simulink model "ExtensionSimulation2CONT"  (R2015b)
settings: Solver=VariableStepAuto  StartTime=0.0  StopTime=60  RelTol=1e-3
values from neighbouring files (symbols this model uses):
  beta_str = 0.5*ones(1,10)    [PlotChannelCont.m]
undefined symbols (not defined in the file or in its folder): alpha_str, MemoryGain, nu_pc, sigbuilder_block, teta, w_e, w_g, w_minus, w_pc, w_plus, w_s, w_t
libraries: fuzblock x35, simulink x1
settings Model: Creator=acaso  LastModifiedBy=acaso

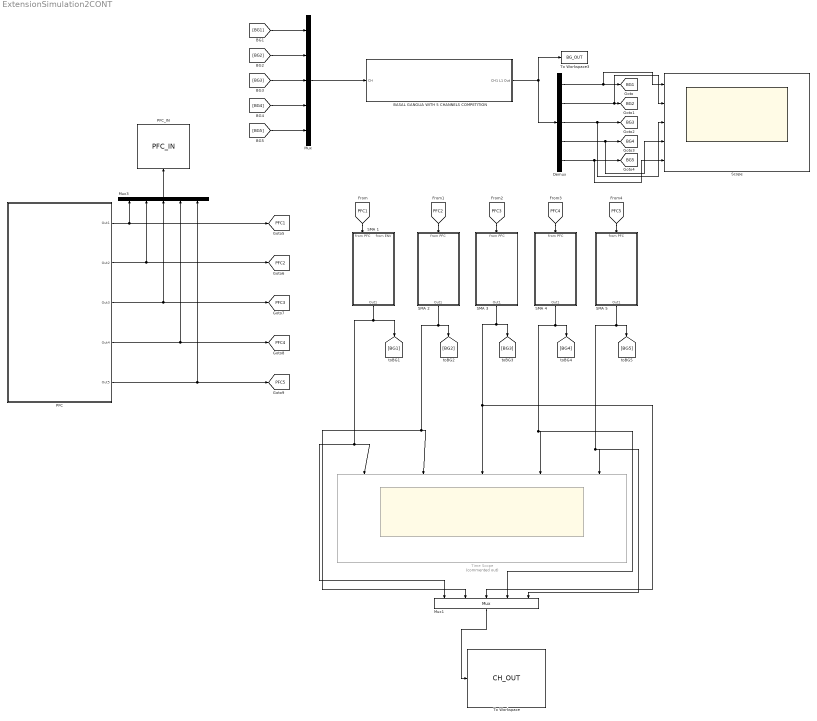
== system ExtensionSimulation2CONT ==
  BASAL GANGLIA WITH 5 CHANNELS COMPETITION : Subsystem
  Demux : Demux  Outputs=5
  Mux : Mux  Inputs=5
  Mux1 : Mux  Inputs=5
  Mux3 : Mux  Inputs=5
  "PFC " : Subsystem
  PFC_IN : ToWorkspace  VariableName=PFC_IN  SaveFormat=Timeseries  SampleTime=0.1
  SMA 1 : Subsystem
  SMA 2 : Subsystem
  SMA 3 : Subsystem
  SMA 4 : Subsystem
  SMA 5 : Subsystem
  Scope : Scope  NumInputPorts=5
  Time Scope : Scope  Commented=on  NumInputPorts=5
  To Workspace : ToWorkspace  VariableName=CH_OUT  SaveFormat=Timeseries  SampleTime=0.1
  To Workspace3 : ToWorkspace  VariableName=BG_OUT  SaveFormat=Timeseries  SampleTime=-1
  tag scope: BG1=global, BG2=global, BG3=global, BG4=global, BG5=global, PFC1=global, PFC2=global, PFC3=global, PFC4=global, PFC5=global
  wires:
  SMA 2/1(Out1) -> [BG2], Time Scope/2, Mux1/2
  SMA 3/1(Out1) -> [BG3], Mux1/3, Time Scope/3
  SMA 4/1(Out1) -> [BG4], Mux1/4, Time Scope/4
  SMA 5/1(Out1) -> [BG5], Mux1/5, Time Scope/5
  Mux/1 -> BASAL GANGLIA WITH 5 CHANNELS COMPETITION/1("CH ")
  Mux1/1 -> To Workspace/1
  Demux/1 -> Scope/1, [BG1]
  Demux/2 -> Scope/2, [BG2]
  Demux/3 -> Scope/3, [BG3]
  Demux/4 -> Scope/4, [BG4]
  Demux/5 -> Scope/5, [BG5]
  BASAL GANGLIA WITH 5 CHANNELS COMPETITION/1(CH1 L1 Out) -> To Workspace3/1, Demux/1
  SMA 1/1(Out1) -> [BG1], Time Scope/1, Mux1/1
  Mux3/1 -> PFC_IN/1
  "PFC "/2(Out2) -> [PFC2], Mux3/2
  "PFC "/3(Out3) -> [PFC3], Mux3/3
  "PFC "/4(Out4) -> [PFC4], Mux3/4
  "PFC "/5(Out5) -> [PFC5], Mux3/5
  [PFC1] -> SMA 1/1(from PFC)
  [PFC2] -> SMA 2/1(from PFC)
  [PFC3] -> SMA 3/1(from PFC)
  [PFC4] -> SMA 4/1(from PFC)
  [PFC5] -> SMA 5/1(from PFC)
  "PFC "/1(Out1) -> [PFC1], Mux3/1
  [BG1] -> Mux/1
  [BG2] -> Mux/2
  [BG3] -> Mux/3
  [BG4] -> Mux/4
  [BG5] -> Mux/5

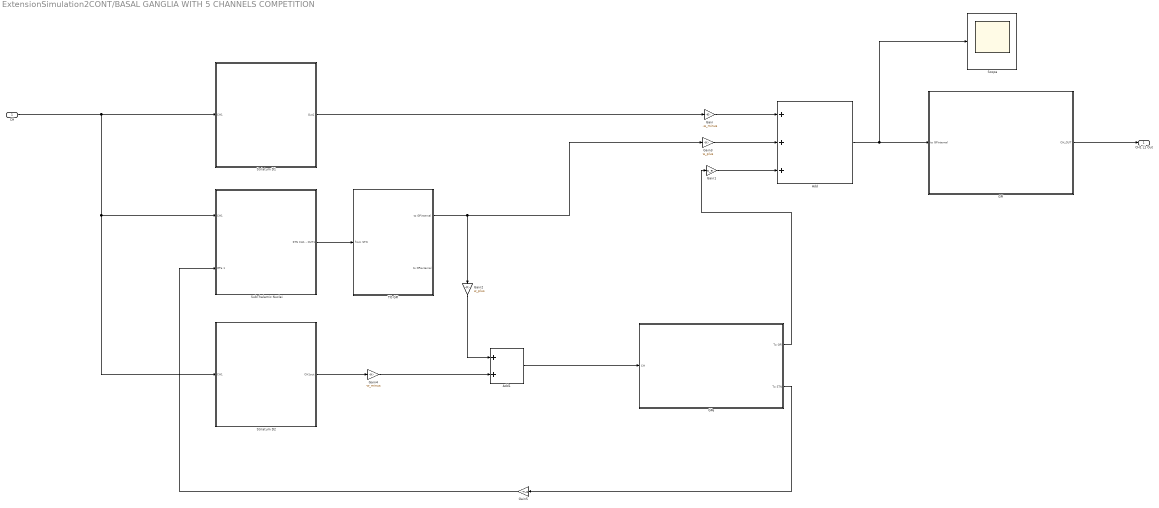
== system ExtensionSimulation2CONT/BASAL GANGLIA WITH 5 CHANNELS COMPETITION ==
  "CH " : Inport
  Add : Sum  Inputs=3
  Add1 : Sum  Inputs=2
  GPe : Subsystem  TreatAsAtomicUnit=on
  GPi : Subsystem
  Gain : Gain  Gain=-w_minus
  Gain1 : Gain  Gain=w_e
  Gain2 : Gain  Gain=w_plus
  Gain3 : Gain  Gain=w_plus
  Gain4 : Gain  Gain=-w_minus
  Gain5 : Gain  Gain=-w_g
  Scope : Scope
  "Striatum D1 " : Subsystem
  Striatum D2 : Subsystem
  SubThalamic Nuclei : Subsystem
  TO GPi : Subsystem
  CH1 L1 Out : Outport
  wires:
  TO GPi/1(to GPinternal) -> Gain3/1, Gain2/1
  GPi/1("CH_OUT ") -> CH1 L1 Out/1
  "CH "/1 -> Striatum D2/1(CH1), SubThalamic Nuclei/1(CH1), "Striatum D1 "/1(CH1)
  "Striatum D1 "/1(Out1) -> Gain/1
  SubThalamic Nuclei/1(STN CH1 - OUT1) -> TO GPi/1("from STN ")
  GPe/1(To GPi) -> Gain1/1
  Gain/1 -> Add/1
  Gain3/1 -> Add/2
  Gain1/1 -> Add/3
  Striatum D2/1(CH1out) -> Gain4/1
  Gain2/1 -> Add1/1
  Gain4/1 -> Add1/2
  Add1/1 -> GPe/1(CH)
  GPe/2(To STN) -> Gain5/1
  Gain5/1 -> SubThalamic Nuclei/2(GPe 1)
  Add/1 -> GPi/1("to GPinternal "), Scope/1

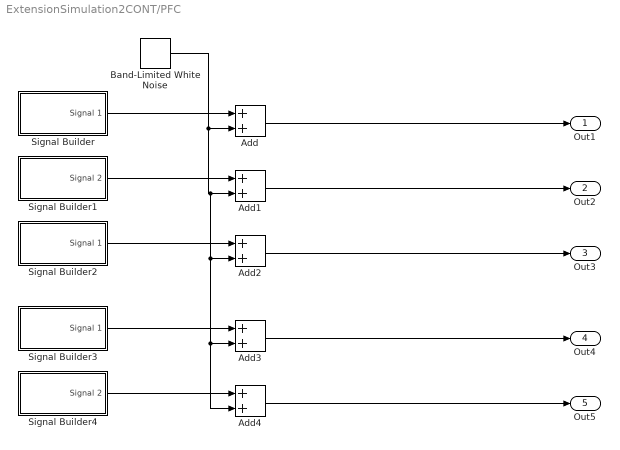
== system ExtensionSimulation2CONT/PFC  ==
  Add{,1..4} (5 alike) : Sum
  Band-Limited White Noise : simulink/Sources/Band-Limited White Noise  Cov=CHNoise  Ts=0.1  seed=[23341]
  Signal Builder : Subsystem  Tag=STV Subsys  LoadFcn=sigbuilder_block('load');  StartFcn=sigbuilder_block('start');  StopFcn=sigbuilder_block('stop');  ClipboardFcn=sigbuilder_block('clipboard');  mask(Sigbuilder block){}
      mask help: Simulink:masks:SigbuilderBlock_MD
      mask init:
      | if ~strcmp(get_param(bdroot(gcbh),'SimulationStatus'),'stopped') tuvar = sigbuilder_block('maskInit'); end
      settings: CopyFcn=sigbuilder_block('copy');  DeleteFcn=sigbuilder_block('delete');  ModelCloseFcn=sigbuilder_block('modelClose');  PreSaveFcn=sigbuilder_block('preSave');  PauseFcn=sigbuilder_block('pause');  ContinueFcn=sigbuilder_block('continue');  NameChangeFcn=sigbuilder_block('namechange');  OpenFcn=sigbuilder_block('open',[428 151 550 399 ]);  CloseFcn=sigbuilder_block('close');
      mask Display: plot(0, 0, 100, 100,[2, 2, 32, 32, 2], [68, 8, 8, 68, 68],[32, 2], [38, 38], [32, 19, 2],[53, 60, 44], [32, 17, 17, 2],[16, 16, 31, 31]);txt = getActiveGroup(gcbh);text(2, 100, txt,'verticalAlignment', 'top');
  Signal Builder1 : Subsystem  Tag=STV Subsys  LoadFcn=sigbuilder_block('load');  StartFcn=sigbuilder_block('start');  StopFcn=sigbuilder_block('stop');  ClipboardFcn=sigbuilder_block('clipboard');  mask(Sigbuilder block){}
      mask help: Simulink:masks:SigbuilderBlock_MD
      mask init:
      | if ~strcmp(get_param(bdroot(gcbh),'SimulationStatus'),'stopped') tuvar = sigbuilder_block('maskInit'); end
      settings: CopyFcn=sigbuilder_block('copy');  DeleteFcn=sigbuilder_block('delete');  ModelCloseFcn=sigbuilder_block('modelClose');  PreSaveFcn=sigbuilder_block('preSave');  PauseFcn=sigbuilder_block('pause');  ContinueFcn=sigbuilder_block('continue');  NameChangeFcn=sigbuilder_block('namechange');  OpenFcn=sigbuilder_block('open',[428 151 550 399 ]);  CloseFcn=sigbuilder_block('close');
      mask Display: plot(0, 0, 100, 100,[2, 2, 32, 32, 2], [68, 8, 8, 68, 68],[32, 2], [38, 38], [32, 19, 2],[53, 60, 44], [32, 17, 17, 2],[16, 16, 31, 31]);txt = getActiveGroup(gcbh);text(2, 100, txt,'verticalAlignment', 'top');
  Signal Builder2 : Subsystem  Tag=STV Subsys  LoadFcn=sigbuilder_block('load');  StartFcn=sigbuilder_block('start');  StopFcn=sigbuilder_block('stop');  ClipboardFcn=sigbuilder_block('clipboard');  mask(Sigbuilder block){}
      mask help: Simulink:masks:SigbuilderBlock_MD
      mask init:
      | if ~strcmp(get_param(bdroot(gcbh),'SimulationStatus'),'stopped') tuvar = sigbuilder_block('maskInit'); end
      settings: CopyFcn=sigbuilder_block('copy');  DeleteFcn=sigbuilder_block('delete');  ModelCloseFcn=sigbuilder_block('modelClose');  PreSaveFcn=sigbuilder_block('preSave');  PauseFcn=sigbuilder_block('pause');  ContinueFcn=sigbuilder_block('continue');  NameChangeFcn=sigbuilder_block('namechange');  OpenFcn=sigbuilder_block('open',[428 151 550 399 ]);  CloseFcn=sigbuilder_block('close');
      mask Display: plot(0, 0, 100, 100,[2, 2, 32, 32, 2], [68, 8, 8, 68, 68],[32, 2], [38, 38], [32, 19, 2],[53, 60, 44], [32, 17, 17, 2],[16, 16, 31, 31]);txt = getActiveGroup(gcbh);text(2, 100, txt,'verticalAlignment', 'top');
  Signal Builder3 : Subsystem  Tag=STV Subsys  LoadFcn=sigbuilder_block('load');  StartFcn=sigbuilder_block('start');  StopFcn=sigbuilder_block('stop');  ClipboardFcn=sigbuilder_block('clipboard');  mask(Sigbuilder block){}
      mask help: Simulink:masks:SigbuilderBlock_MD
      mask init:
      | if ~strcmp(get_param(bdroot(gcbh),'SimulationStatus'),'stopped') tuvar = sigbuilder_block('maskInit'); end
      settings: CopyFcn=sigbuilder_block('copy');  DeleteFcn=sigbuilder_block('delete');  ModelCloseFcn=sigbuilder_block('modelClose');  PreSaveFcn=sigbuilder_block('preSave');  PauseFcn=sigbuilder_block('pause');  ContinueFcn=sigbuilder_block('continue');  NameChangeFcn=sigbuilder_block('namechange');  OpenFcn=sigbuilder_block('open',[428 151 550 399 ]);  CloseFcn=sigbuilder_block('close');
      mask Display: plot(0, 0, 100, 100,[2, 2, 32, 32, 2], [68, 8, 8, 68, 68],[32, 2], [38, 38], [32, 19, 2],[53, 60, 44], [32, 17, 17, 2],[16, 16, 31, 31]);txt = getActiveGroup(gcbh);text(2, 100, txt,'verticalAlignment', 'top');
  Signal Builder4 : Subsystem  Tag=STV Subsys  LoadFcn=sigbuilder_block('load');  StartFcn=sigbuilder_block('start');  StopFcn=sigbuilder_block('stop');  ClipboardFcn=sigbuilder_block('clipboard');  mask(Sigbuilder block){}
      mask help: Simulink:masks:SigbuilderBlock_MD
      mask init:
      | if ~strcmp(get_param(bdroot(gcbh),'SimulationStatus'),'stopped') tuvar = sigbuilder_block('maskInit'); end
      settings: CopyFcn=sigbuilder_block('copy');  DeleteFcn=sigbuilder_block('delete');  ModelCloseFcn=sigbuilder_block('modelClose');  PreSaveFcn=sigbuilder_block('preSave');  PauseFcn=sigbuilder_block('pause');  ContinueFcn=sigbuilder_block('continue');  NameChangeFcn=sigbuilder_block('namechange');  OpenFcn=sigbuilder_block('open',[428 151 550 399 ]);  CloseFcn=sigbuilder_block('close');
      mask Display: plot(0, 0, 100, 100,[2, 2, 32, 32, 2], [68, 8, 8, 68, 68],[32, 2], [38, 38], [32, 19, 2],[53, 60, 44], [32, 17, 17, 2],[16, 16, 31, 31]);txt = getActiveGroup(gcbh);text(2, 100, txt,'verticalAlignment', 'top');
  Out1 : Outport
  Out2 : Outport  Port=2
  Out3 : Outport  Port=3
  Out4 : Outport  Port=4
  Out5 : Outport  Port=5
  wires:
  Signal Builder/1(Signal 1) -> Add/1
  Add/1 -> Out1/1
  Signal Builder1/1(Signal 2) -> Add1/1
  Add1/1 -> Out2/1
  Add2/1 -> Out3/1
  Signal Builder4/1(Signal 2) -> Add4/1
  Add4/1 -> Out5/1
  Add3/1 -> Out4/1
  Band-Limited White Noise/1 -> Add4/2, Add3/2, Add2/2, Add1/2, Add/2
  Signal Builder3/1(Signal 1) -> Add3/1
  Signal Builder2/1(Signal 1) -> Add2/1

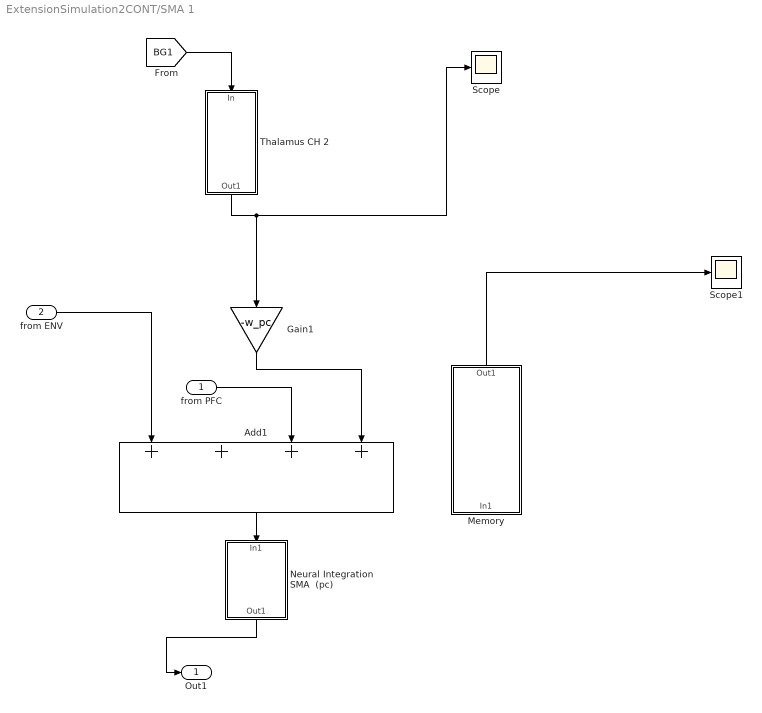
== system ExtensionSimulation2CONT/SMA 1 ==
  from PFC : Inport
  "from ENV " : Inport  Port=2
  Add1 : Sum  Inputs=4
  Gain1 : Gain  Gain=-w_pc
  Memory : Subsystem
  Neural Integration SMA  (pc) : Subsystem
  Scope : Scope
  Scope1 : Scope
  Thalamus CH 2 : Subsystem
  Out1 : Outport
  wires:
  from PFC/1 -> Add1/3
  Add1/1 -> Neural Integration SMA  (pc)/1(In1)
  [BG1] -> Thalamus CH 2/1("In ")
  Gain1/1 -> Add1/4
  Thalamus CH 2/1(Out1) -> Scope/1, Gain1/1
  Neural Integration SMA  (pc)/1(Out1) -> Out1/1
  Memory/1(Out1) -> Scope1/1
  "from ENV "/1 -> Add1/1

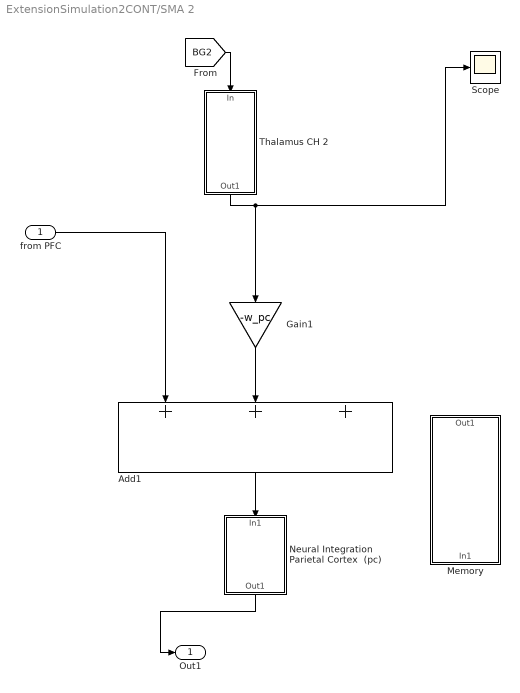
== system ExtensionSimulation2CONT/SMA 2 ==
  from PFC : Inport
  Add1 : Sum  Inputs=3
  Gain1 : Gain  Gain=-w_pc
  Memory : Subsystem
  Neural Integration Parietal Cortex  (pc) : Subsystem
  Scope : Scope
  Thalamus CH 2 : Subsystem
  Out1 : Outport
  wires:
  from PFC/1 -> Add1/1
  Add1/1 -> Neural Integration Parietal Cortex  (pc)/1(In1)
  [BG2] -> Thalamus CH 2/1("In ")
  Gain1/1 -> Add1/2
  Thalamus CH 2/1(Out1) -> Scope/1, Gain1/1
  Neural Integration Parietal Cortex  (pc)/1(Out1) -> Out1/1

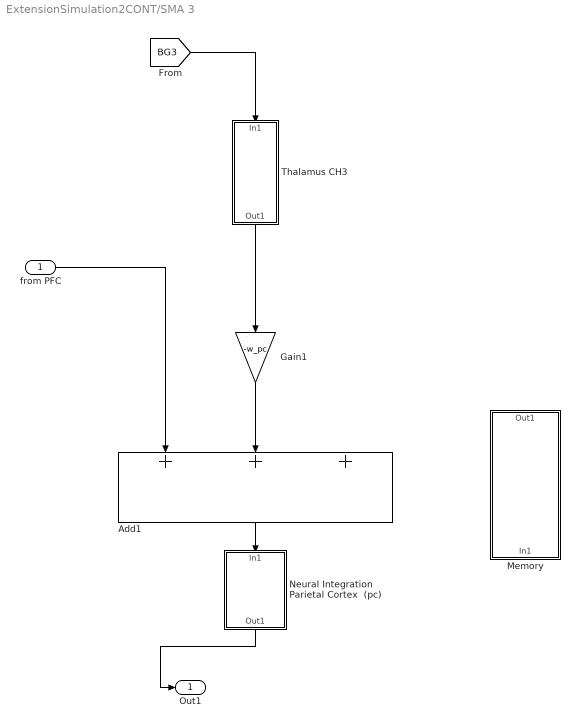
== system ExtensionSimulation2CONT/SMA 3 ==
  from PFC : Inport
  Add1 : Sum  Inputs=3
  Gain1 : Gain  Gain=-w_pc
  Memory : Subsystem
  Neural Integration Parietal Cortex  (pc) : Subsystem
  "Thalamus CH3 " : Subsystem
  Out1 : Outport
  wires:
  from PFC/1 -> Add1/1
  Add1/1 -> Neural Integration Parietal Cortex  (pc)/1(In1)
  Neural Integration Parietal Cortex  (pc)/1(Out1) -> Out1/1
  [BG3] -> "Thalamus CH3 "/1(In1)
  "Thalamus CH3 "/1(Out1) -> Gain1/1
  Gain1/1 -> Add1/2

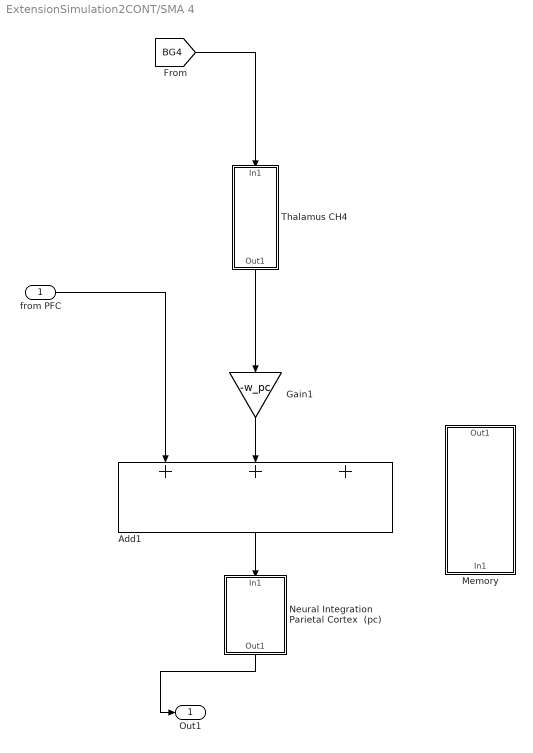
== system ExtensionSimulation2CONT/SMA 4 ==
  from PFC : Inport
  Add1 : Sum  Inputs=3
  Gain1 : Gain  Gain=-w_pc
  Memory : Subsystem
  Neural Integration Parietal Cortex  (pc) : Subsystem
  "Thalamus CH4 " : Subsystem
  Out1 : Outport
  wires:
  from PFC/1 -> Add1/1
  Add1/1 -> Neural Integration Parietal Cortex  (pc)/1(In1)
  Neural Integration Parietal Cortex  (pc)/1(Out1) -> Out1/1
  [BG4] -> "Thalamus CH4 "/1(In1)
  "Thalamus CH4 "/1(Out1) -> Gain1/1
  Gain1/1 -> Add1/2

== system ExtensionSimulation2CONT/SMA 5 ==
  from PFC : Inport
  Add1 : Sum  Inputs=3
  Gain1 : Gain  Gain=-w_pc
  Memory : Subsystem
  Neural Integration Parietal Cortex  (pc) : Subsystem
  "Thalamus CH5 " : Subsystem
  Out1 : Outport
  wires:
  from PFC/1 -> Add1/1
  Add1/1 -> Neural Integration Parietal Cortex  (pc)/1(In1)
  Neural Integration Parietal Cortex  (pc)/1(Out1) -> Out1/1
  [BG5] -> "Thalamus CH5 "/1(In1)
  "Thalamus CH5 "/1(Out1) -> Gain1/1
  Gain1/1 -> Add1/2

== system ExtensionSimulation2CONT/BASAL GANGLIA WITH 5 CHANNELS COMPETITION/GPe ==
  CH : Inport
  GPe CH1 : Subsystem
  To GPi : Outport
  To STN : Outport  Port=2
  wires:
  CH/1 -> GPe CH1/1(In)
  GPe CH1/1(To GPi) -> To GPi/1
  GPe CH1/2(To STN) -> To STN/1

== system ExtensionSimulation2CONT/BASAL GANGLIA WITH 5 CHANNELS COMPETITION/GPi ==
  "to GPinternal " : Inport
  GPinternal : Subsystem
  "CH_OUT " : Outport
  wires:
  "to GPinternal "/1 -> GPinternal/1("to GPinternal ")
  GPinternal/1(To Thal) -> "CH_OUT "/1

== system ExtensionSimulation2CONT/BASAL GANGLIA WITH 5 CHANNELS COMPETITION/Striatum D1  ==
  CH1 : Inport
  "Striatum D1 " : Subsystem
  Out1 : Outport
  wires:
  CH1/1 -> "Striatum D1 "/1(Channel)
  "Striatum D1 "/1(Striatum D1 Out) -> Out1/1

== system ExtensionSimulation2CONT/BASAL GANGLIA WITH 5 CHANNELS COMPETITION/Striatum D2 ==
  CH1 : Inport
  Scope : Scope
  "Striatum D2 " : Subsystem
  CH1out : Outport
  wires:
  "Striatum D2 "/1(Striatum D1 Out) -> Scope/1, CH1out/1
  CH1/1 -> "Striatum D2 "/1(Channel)

== system ExtensionSimulation2CONT/BASAL GANGLIA WITH 5 CHANNELS COMPETITION/SubThalamic Nuclei ==
  CH1 : Inport
  GPe 1 : Inport  Port=2
  "SubThalamic Nucleus (STN) " : Subsystem
  STN CH1 - OUT1 : Outport
  wires:
  CH1/1 -> "SubThalamic Nucleus (STN) "/1(Channel)
  GPe 1/1 -> "SubThalamic Nucleus (STN) "/2(GPe Inp)
  "SubThalamic Nucleus (STN) "/1(STN Out1) -> STN CH1 - OUT1/1

== system ExtensionSimulation2CONT/BASAL GANGLIA WITH 5 CHANNELS COMPETITION/TO GPi ==
  "from STN " : Inport
  Add : Sum  Inputs=5
  Demux : Demux  Outputs=5
  Mux : Mux  Inputs=5
  Scope : Scope
  Scope1 : Scope
  to GPinternal : Outport
  to GPexternal : Outport  Port=2
  wires:
  "from STN "/1 -> Scope/1, Demux/1
  Demux/1 -> Add/1
  Demux/2 -> Add/2
  Demux/3 -> Add/3
  Demux/4 -> Add/4
  Demux/5 -> Add/5
  Add/1 -> Scope1/1, Mux/1, Mux/2, Mux/3, Mux/4, Mux/5
  Mux/1 -> to GPexternal/1, to GPinternal/1

== system ExtensionSimulation2CONT/PFC /Signal Builder ==
  Demux : Demux  Tag=STV Demux  Outputs=1
  FromWs : FromWorkspace  Tag=STV FromWs  VariableName=tuvar  SampleTime=0
      SigBuilderData=|
      | common.afterFinalStr = 'Extrapolate'
      | common.sampleTime = 0
      | dataSet.timeRange = [0 60]
      | dataSet.name = 'Group 1'
      | sbobj.Groups.Name = 'Group 1'
      | sbobj.Groups.Signals.Name = 'Signal 1'
      | sbobj.Groups.Signals.XData = [0 9.8 9.8 30 30 60]
      | sbobj.Groups.Signals.YData = [0 0 0.985 0.985 0 0]
      | sbobj.Groups.TimeRange = [0 60]
  Signal 1 : Outport  Tag=STV Outport
  wires:
  Demux/1 -> Signal 1/1
  FromWs/1 -> Demux/1

== system ExtensionSimulation2CONT/PFC /Signal Builder1 ==
  Demux : Demux  Tag=STV Demux  Outputs=1
  FromWs : FromWorkspace  Tag=STV FromWs  VariableName=tuvar  SampleTime=0
      SigBuilderData=|
      | common.afterFinalStr = 'Extrapolate'
      | common.sampleTime = 0
      | dataSet.timeRange = [0 60]
      | dataSet.name = 'Group 1'
      | sbobj.Groups.Name = 'Group 1'
      | sbobj.Groups.Signals.Name = 'Signal 2'
      | sbobj.Groups.Signals.XData = [0 19.8 19.8 39.8 39.8 60]
      | sbobj.Groups.Signals.YData = [0 0 0.98 0.98 0 0]
      | sbobj.Groups.TimeRange = [0 60]
  Signal 2 : Outport  Tag=STV Outport
  wires:
  FromWs/1 -> Demux/1
  Demux/1 -> Signal 2/1

== system ExtensionSimulation2CONT/PFC /Signal Builder2 ==
  Demux : Demux  Tag=STV Demux  Outputs=1
  FromWs : FromWorkspace  Tag=STV FromWs  VariableName=tuvar  SampleTime=0
      SigBuilderData=|
      | common.afterFinalStr = 'Extrapolate'
      | common.sampleTime = 0
      | dataSet.timeRange = [0 60]
      | dataSet.name = 'Group 1'
      | sbobj.Groups.Name = 'Group 1'
      | sbobj.Groups.Signals.Name = 'Signal 1'
      | sbobj.Groups.Signals.XData = [0 30 30 40 40 60]
      | sbobj.Groups.Signals.YData = [0 0 1 1 0 0]
      | sbobj.Groups.TimeRange = [0 60]
  Signal 1 : Outport  Tag=STV Outport
  wires:
  FromWs/1 -> Demux/1
  Demux/1 -> Signal 1/1

== system ExtensionSimulation2CONT/PFC /Signal Builder3 ==
  Demux : Demux  Tag=STV Demux  Outputs=1
  FromWs : FromWorkspace  Tag=STV FromWs  VariableName=tuvar  SampleTime=0
      SigBuilderData=|
      | common.afterFinalStr = 'Extrapolate'
      | common.sampleTime = 0
      | dataSet.timeRange = [0 60]
      | dataSet.name = 'Group 1'
      | sbobj.Groups.Name = 'Group 1'
      | sbobj.Groups.Signals.Name = 'Signal 1'
      | sbobj.Groups.Signals.XData = [0 40 40 50.2 50.2 60]
      | sbobj.Groups.Signals.YData = [0 0 1 1 0 0]
      | sbobj.Groups.TimeRange = [0 60]
  Signal 1 : Outport  Tag=STV Outport
  wires:
  FromWs/1 -> Demux/1
  Demux/1 -> Signal 1/1

== system ExtensionSimulation2CONT/PFC /Signal Builder4 ==
  Demux : Demux  Tag=STV Demux  Outputs=1
  FromWs : FromWorkspace  Tag=STV FromWs  VariableName=tuvar  SampleTime=0
      SigBuilderData=|
      | common.afterFinalStr = 'Extrapolate'
      | common.sampleTime = 0
      | dataSet.timeRange = [0 10]
      | dataSet.name = 'Group 1'
      | sbobj.Groups.Name = 'Group 1'
      | sbobj.Groups.Signals.Name = 'Signal 2'
      | sbobj.Groups.Signals.XData = [0 10]
      | sbobj.Groups.Signals.YData = [0.08 0.08]
  Signal 2 : Outport  Tag=STV Outport
  wires:
  FromWs/1 -> Demux/1
  Demux/1 -> Signal 2/1

== system ExtensionSimulation2CONT/SMA 1/Memory ==
  In1 : Inport
  "Leaky-Integrator Striatum D1 " : ZeroPole  Zeros=[]  Poles=[-1]
  "MemoryGain " : Gain  Gain=MemoryGain
  Scope1 : Scope  NumInputPorts=2
  Self-Resetting System : Subsystem
  Out1 : Outport
  wires:
  "Leaky-Integrator Striatum D1 "/1 -> "MemoryGain "/1
  "MemoryGain "/1 -> Scope1/1, Out1/1
  In1/1 -> Scope1/2, Self-Resetting System/1(In1)
  Self-Resetting System/1(Out1) -> "Leaky-Integrator Striatum D1 "/1

== system ExtensionSimulation2CONT/SMA 1/Neural Integration SMA  (pc) ==
  In1 : Inport
  "Leaky-Integrator Striatum D1 " : ZeroPole  Zeros=[]  Poles=[-1/teta]  Gain=[1.5/teta]
  Sigmoidal MF : fuzblock/Membership  Functions/Sigmoidal MF  a=alpha_pc  c=beta_pc
  Out1 : Outport
  wires:
  In1/1 -> "Leaky-Integrator Striatum D1 "/1
  "Leaky-Integrator Striatum D1 "/1 -> Sigmoidal MF/1
  Sigmoidal MF/1 -> Out1/1

== system ExtensionSimulation2CONT/SMA 1/Thalamus CH 2 ==
  "In " : Inport
  Neural Integration Thalamus  (pc) : Subsystem
  Out1 : Outport
  wires:
  Neural Integration Thalamus  (pc)/1(Out1) -> Out1/1
  "In "/1 -> Neural Integration Thalamus  (pc)/1(In1)

== system ExtensionSimulation2CONT/SMA 2/Memory ==
  In1 : Inport
  "Leaky-Integrator Striatum D1 " : ZeroPole  Zeros=[]  Poles=[-1]
  "MemoryGain " : Gain  Gain=MemoryGain
  Scope1 : Scope  NumInputPorts=2
  Self-Resetting System : Subsystem
  Out1 : Outport
  wires:
  "Leaky-Integrator Striatum D1 "/1 -> "MemoryGain "/1
  "MemoryGain "/1 -> Scope1/1, Out1/1
  In1/1 -> Scope1/2, Self-Resetting System/1(In1)
  Self-Resetting System/1(Out1) -> "Leaky-Integrator Striatum D1 "/1

== system ExtensionSimulation2CONT/SMA 2/Neural Integration Parietal Cortex  (pc) ==
  In1 : Inport
  Fcn : Fcn  Expr=u^(1/nu_pc)
  "Leaky-Integrator Striatum D1 " : ZeroPole  Zeros=[]  Poles=[-1/teta]  Gain=[1.5/teta]
  Sigmoidal MF : fuzblock/Membership  Functions/Sigmoidal MF  a=alpha_pc  c=beta_pc
  Out1 : Outport
  wires:
  In1/1 -> "Leaky-Integrator Striatum D1 "/1
  Sigmoidal MF/1 -> Fcn/1
  "Leaky-Integrator Striatum D1 "/1 -> Sigmoidal MF/1
  Fcn/1 -> Out1/1

== system ExtensionSimulation2CONT/SMA 2/Thalamus CH 2 ==
  "In " : Inport
  Neural Integration Thalamus  (pc) : Subsystem
  Out1 : Outport
  wires:
  Neural Integration Thalamus  (pc)/1(Out1) -> Out1/1
  "In "/1 -> Neural Integration Thalamus  (pc)/1(In1)

== system ExtensionSimulation2CONT/SMA 3/Memory ==
  In1 : Inport
  "Leaky-Integrator Striatum D1 " : ZeroPole  Zeros=[]  Poles=[-1]
  "MemoryGain " : Gain  Gain=MemoryGain
  Scope1 : Scope  NumInputPorts=2
  Self-Resetting System : Subsystem
  Out1 : Outport
  wires:
  "Leaky-Integrator Striatum D1 "/1 -> "MemoryGain "/1
  "MemoryGain "/1 -> Scope1/1, Out1/1
  In1/1 -> Scope1/2, Self-Resetting System/1(In1)
  Self-Resetting System/1(Out1) -> "Leaky-Integrator Striatum D1 "/1

== system ExtensionSimulation2CONT/SMA 3/Neural Integration Parietal Cortex  (pc) ==
  In1 : Inport
  Fcn : Fcn  Expr=u^(1/nu_pc)
  "Leaky-Integrator Striatum D1 " : ZeroPole  Zeros=[]  Poles=[-1/teta]  Gain=[1.5/teta]
  Sigmoidal MF : fuzblock/Membership  Functions/Sigmoidal MF  a=alpha_pc  c=beta_pc
  Out1 : Outport
  wires:
  In1/1 -> "Leaky-Integrator Striatum D1 "/1
  Sigmoidal MF/1 -> Fcn/1
  "Leaky-Integrator Striatum D1 "/1 -> Sigmoidal MF/1
  Fcn/1 -> Out1/1

== system ExtensionSimulation2CONT/SMA 3/Thalamus CH3  ==
  In1 : Inport
  Neural Integration Thalamus  (pc) : Subsystem
  Out1 : Outport
  wires:
  Neural Integration Thalamus  (pc)/1(Out1) -> Out1/1
  In1/1 -> Neural Integration Thalamus  (pc)/1(In1)

== system ExtensionSimulation2CONT/SMA 4/Memory ==
  In1 : Inport
  "Leaky-Integrator Striatum D1 " : ZeroPole  Zeros=[]  Poles=[-1]
  "MemoryGain " : Gain  Gain=MemoryGain
  Scope1 : Scope  NumInputPorts=2
  Self-Resetting System : Subsystem
  Out1 : Outport
  wires:
  "Leaky-Integrator Striatum D1 "/1 -> "MemoryGain "/1
  "MemoryGain "/1 -> Scope1/1, Out1/1
  In1/1 -> Scope1/2, Self-Resetting System/1(In1)
  Self-Resetting System/1(Out1) -> "Leaky-Integrator Striatum D1 "/1

== system ExtensionSimulation2CONT/SMA 4/Neural Integration Parietal Cortex  (pc) ==
  In1 : Inport
  Fcn : Fcn  Expr=u^(1/nu_pc)
  "Leaky-Integrator Striatum D1 " : ZeroPole  Zeros=[]  Poles=[-1/teta]  Gain=[1.5/teta]
  Sigmoidal MF : fuzblock/Membership  Functions/Sigmoidal MF  a=alpha_pc  c=beta_pc
  Out1 : Outport
  wires:
  In1/1 -> "Leaky-Integrator Striatum D1 "/1
  Sigmoidal MF/1 -> Fcn/1
  "Leaky-Integrator Striatum D1 "/1 -> Sigmoidal MF/1
  Fcn/1 -> Out1/1

== system ExtensionSimulation2CONT/SMA 4/Thalamus CH4  ==
  In1 : Inport
  Neural Integration Thalamus  (pc) : Subsystem
  Thalamic activation : Fcn  Expr=(1 - u)
  Out1 : Outport
  wires:
  Neural Integration Thalamus  (pc)/1(Out1) -> Out1/1
  In1/1 -> Neural Integration Thalamus  (pc)/1(In1)

== system ExtensionSimulation2CONT/SMA 5/Memory ==
  In1 : Inport
  "Leaky-Integrator Striatum D1 " : ZeroPole  Zeros=[]  Poles=[-1]
  "MemoryGain " : Gain  Gain=MemoryGain
  Scope1 : Scope  NumInputPorts=2
  Self-Resetting System : Subsystem
  Out1 : Outport
  wires:
  "Leaky-Integrator Striatum D1 "/1 -> "MemoryGain "/1
  "MemoryGain "/1 -> Scope1/1, Out1/1
  In1/1 -> Scope1/2, Self-Resetting System/1(In1)
  Self-Resetting System/1(Out1) -> "Leaky-Integrator Striatum D1 "/1

== system ExtensionSimulation2CONT/SMA 5/Neural Integration Parietal Cortex  (pc) ==
  In1 : Inport
  Fcn : Fcn  Expr=u^(1/nu_pc)
  "Leaky-Integrator Striatum D1 " : ZeroPole  Zeros=[]  Poles=[-1/teta]  Gain=[1.5/teta]
  Sigmoidal MF : fuzblock/Membership  Functions/Sigmoidal MF  a=alpha_pc  c=beta_pc
  Out1 : Outport
  wires:
  In1/1 -> "Leaky-Integrator Striatum D1 "/1
  Sigmoidal MF/1 -> Fcn/1
  "Leaky-Integrator Striatum D1 "/1 -> Sigmoidal MF/1
  Fcn/1 -> Out1/1

== system ExtensionSimulation2CONT/SMA 5/Thalamus CH5  ==
  In1 : Inport
  Neural Integration Thalamus  (pc) : Subsystem
  Out1 : Outport
  wires:
  Neural Integration Thalamus  (pc)/1(Out1) -> Out1/1
  In1/1 -> Neural Integration Thalamus  (pc)/1(In1)

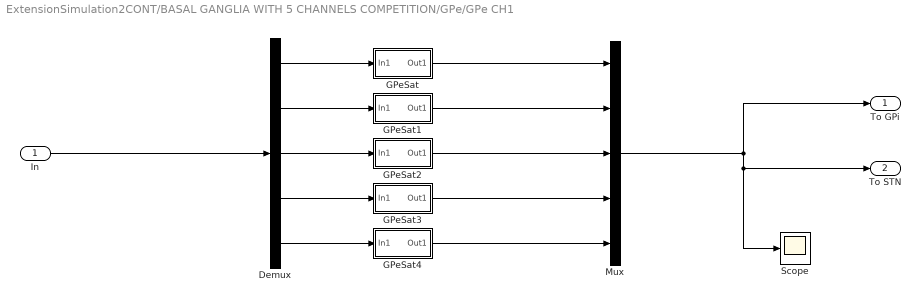
== system ExtensionSimulation2CONT/BASAL GANGLIA WITH 5 CHANNELS COMPETITION/GPe/GPe CH1 ==
  In : Inport
  Demux : Demux  Outputs=5
  GPeSat : Subsystem
  GPeSat1 : Subsystem
  GPeSat2 : Subsystem
  GPeSat3 : Subsystem
  GPeSat4 : Subsystem
  Mux : Mux  Inputs=5
  Scope : Scope
  To GPi : Outport
  To STN : Outport  Port=2
  wires:
  Mux/1 -> To STN/1, Scope/1, To GPi/1
  Demux/1 -> GPeSat/1(In1)
  GPeSat/1(Out1) -> Mux/1
  Demux/2 -> GPeSat1/1(In1)
  GPeSat1/1(Out1) -> Mux/2
  Demux/3 -> GPeSat2/1(In1)
  GPeSat2/1(Out1) -> Mux/3
  Demux/4 -> GPeSat3/1(In1)
  GPeSat3/1(Out1) -> Mux/4
  Demux/5 -> GPeSat4/1(In1)
  GPeSat4/1(Out1) -> Mux/5
  In/1 -> Demux/1

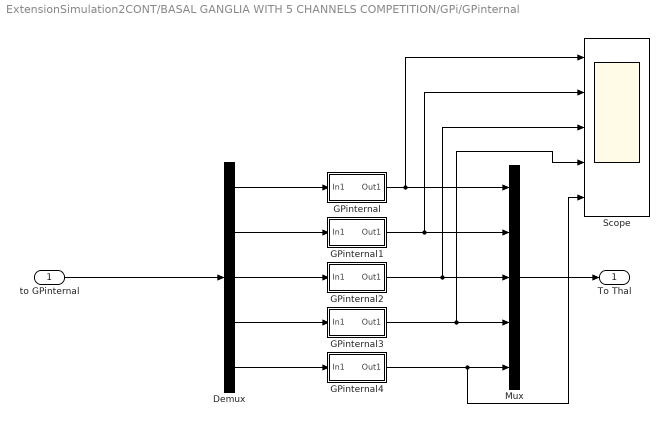
== system ExtensionSimulation2CONT/BASAL GANGLIA WITH 5 CHANNELS COMPETITION/GPi/GPinternal ==
  "to GPinternal " : Inport
  Demux : Demux  Outputs=5
  GPinternal : Subsystem
  GPinternal1 : Subsystem
  GPinternal2 : Subsystem
  GPinternal3 : Subsystem
  GPinternal4 : Subsystem
  Mux : Mux  Inputs=5
  Scope : Scope  NumInputPorts=5
  To Thal : Outport
  wires:
  Demux/1 -> GPinternal/1(In1)
  GPinternal/1(Out1) -> Mux/1, Scope/1
  Demux/2 -> GPinternal1/1(In1)
  Demux/3 -> GPinternal2/1(In1)
  GPinternal2/1(Out1) -> Scope/3, Mux/3
  Demux/4 -> GPinternal3/1(In1)
  GPinternal3/1(Out1) -> Scope/4, Mux/4
  Demux/5 -> GPinternal4/1(In1)
  GPinternal4/1(Out1) -> Scope/5, Mux/5
  "to GPinternal "/1 -> Demux/1
  Mux/1 -> To Thal/1
  GPinternal1/1(Out1) -> Scope/2, Mux/2

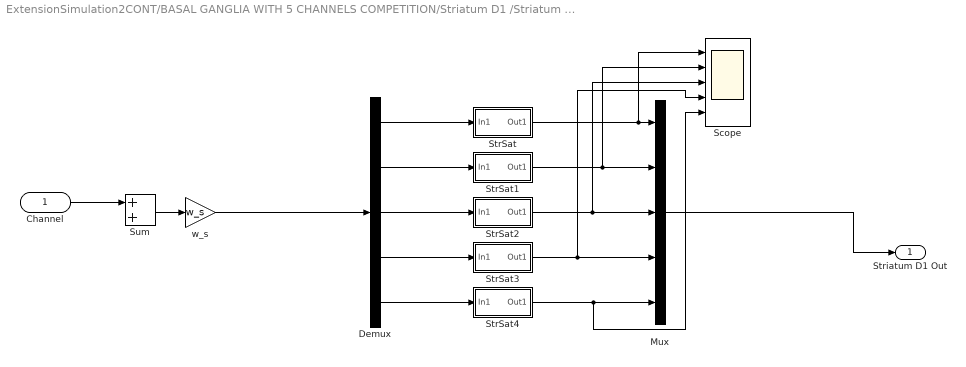
== system ExtensionSimulation2CONT/BASAL GANGLIA WITH 5 CHANNELS COMPETITION/Striatum D1 /Striatum D1  ==
  Channel : Inport
  Demux : Demux  Outputs=5
  Mux : Mux  Inputs=5
  Scope : Scope  NumInputPorts=5
  StrSat : Subsystem
  StrSat1 : Subsystem
  StrSat2 : Subsystem
  StrSat3 : Subsystem
  StrSat4 : Subsystem
  Sum : Sum
  w_s : Gain  Gain=w_s
  Striatum D1 Out : Outport
  wires:
  Channel/1 -> Sum/1
  Sum/1 -> w_s/1
  Mux/1 -> Striatum D1 Out/1
  Demux/1 -> StrSat/1(In1)
  StrSat/1(Out1) -> Scope/1, Mux/1
  Demux/2 -> StrSat1/1(In1)
  StrSat1/1(Out1) -> Scope/2, Mux/2
  Demux/3 -> StrSat2/1(In1)
  StrSat2/1(Out1) -> Scope/3, Mux/3
  Demux/4 -> StrSat3/1(In1)
  StrSat3/1(Out1) -> Scope/4, Mux/4
  Demux/5 -> StrSat4/1(In1)
  w_s/1 -> Demux/1
  StrSat4/1(Out1) -> Scope/5, Mux/5

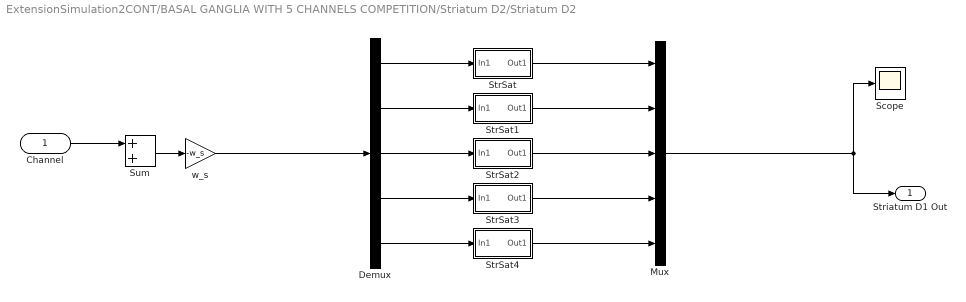
== system ExtensionSimulation2CONT/BASAL GANGLIA WITH 5 CHANNELS COMPETITION/Striatum D2/Striatum D2  ==
  Channel : Inport
  Demux : Demux  Outputs=5
  Mux : Mux  Inputs=5
  Scope : Scope
  StrSat : Subsystem
  StrSat1 : Subsystem
  StrSat2 : Subsystem
  StrSat3 : Subsystem
  StrSat4 : Subsystem
  Sum : Sum
  w_s : Gain  Gain=-w_s
  Striatum D1 Out : Outport
  wires:
  Channel/1 -> Sum/1
  Sum/1 -> w_s/1
  Mux/1 -> Striatum D1 Out/1, Scope/1
  Demux/1 -> StrSat/1(In1)
  StrSat/1(Out1) -> Mux/1
  Demux/2 -> StrSat1/1(In1)
  StrSat1/1(Out1) -> Mux/2
  Demux/3 -> StrSat2/1(In1)
  StrSat2/1(Out1) -> Mux/3
  Demux/4 -> StrSat3/1(In1)
  StrSat3/1(Out1) -> Mux/4
  Demux/5 -> StrSat4/1(In1)
  StrSat4/1(Out1) -> Mux/5
  w_s/1 -> Demux/1

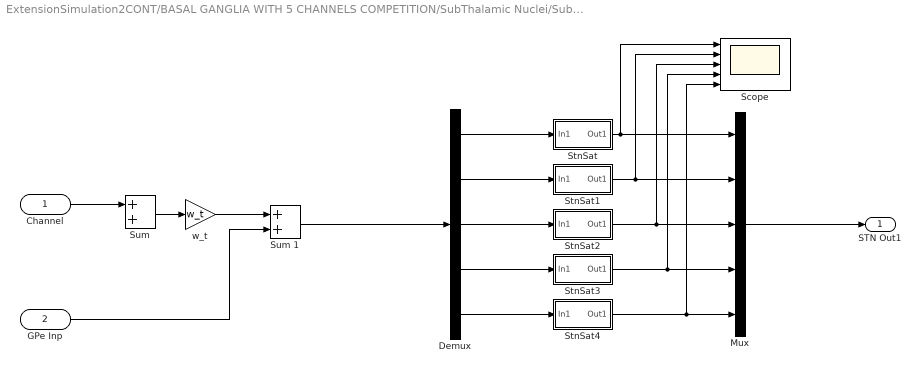
== system ExtensionSimulation2CONT/BASAL GANGLIA WITH 5 CHANNELS COMPETITION/SubThalamic Nuclei/SubThalamic Nucleus (STN)  ==
  Channel : Inport
  GPe Inp : Inport  Port=2
  Demux : Demux  Outputs=5
  Mux : Mux  Inputs=5
  Scope : Scope  NumInputPorts=5
  StnSat : Subsystem
  StnSat1 : Subsystem
  StnSat2 : Subsystem
  StnSat3 : Subsystem
  StnSat4 : Subsystem
  "Sum " : Sum
  Sum 1 : Sum
  w_t : Gain  Gain=w_t
  STN Out1 : Outport
  wires:
  w_t/1 -> Sum 1/1
  Channel/1 -> "Sum "/1
  "Sum "/1 -> w_t/1
  GPe Inp/1 -> Sum 1/2
  Mux/1 -> STN Out1/1
  Demux/1 -> StnSat/1(In1)
  Demux/2 -> StnSat1/1(In1)
  StnSat1/1(Out1) -> Scope/2, Mux/2
  Demux/3 -> StnSat2/1(In1)
  StnSat2/1(Out1) -> Scope/3, Mux/3
  Demux/4 -> StnSat3/1(In1)
  StnSat3/1(Out1) -> Scope/4, Mux/4
  Demux/5 -> StnSat4/1(In1)
  StnSat4/1(Out1) -> Scope/5, Mux/5
  Sum 1/1 -> Demux/1
  StnSat/1(Out1) -> Scope/1, Mux/1

== system ExtensionSimulation2CONT/SMA 1/Memory/Self-Resetting System ==
  In1 : Inport
  Product : Product
  Relay : Relay  OnSwitchValue=MemoryGain  OffSwitchValue=0.1
  Reset Timer : Subsystem
  Saturation : Saturate
  Scope : Scope  NumInputPorts=2
  Out1 : Outport
  wires:
  Relay/1 -> Reset Timer/1(R)
  In1/1 -> Product/2, Scope/1, Relay/1
  Reset Timer/1(Out) -> Product/1
  Product/1 -> Saturation/1
  Saturation/1 -> Out1/1, Scope/2

== system ExtensionSimulation2CONT/SMA 1/Thalamus CH 2/Neural Integration Thalamus  (pc) ==
  In1 : Inport
  "Leaky-Integrator Striatum D1 " : ZeroPole  Zeros=[]  Poles=[-1/teta]  Gain=[1.5/teta]
  Sigmoidal MF : fuzblock/Membership  Functions/Sigmoidal MF  a=alpha_thal  c=beta_thal
  Out1 : Outport
  wires:
  In1/1 -> "Leaky-Integrator Striatum D1 "/1
  "Leaky-Integrator Striatum D1 "/1 -> Sigmoidal MF/1
  Sigmoidal MF/1 -> Out1/1

== system ExtensionSimulation2CONT/SMA 2/Memory/Self-Resetting System ==
  In1 : Inport
  Product : Product
  Relay : Relay  OnSwitchValue=MemoryGain  OffSwitchValue=0.1
  Reset Timer : Subsystem
  Saturation : Saturate
  Scope : Scope  NumInputPorts=2
  Out1 : Outport
  wires:
  Relay/1 -> Reset Timer/1(R)
  In1/1 -> Product/2, Scope/1, Relay/1
  Reset Timer/1(Out) -> Product/1
  Product/1 -> Saturation/1
  Saturation/1 -> Out1/1, Scope/2

== system ExtensionSimulation2CONT/SMA 2/Thalamus CH 2/Neural Integration Thalamus  (pc) ==
  In1 : Inport
  "Leaky-Integrator Striatum D1 " : ZeroPole  Zeros=[]  Poles=[-1/teta]  Gain=[1.5/teta]
  "Sigmoidal Thalamus " : fuzblock/Membership  Functions/Sigmoidal MF  a=alpha_thal  c=beta_thal
  Out1 : Outport
  wires:
  In1/1 -> "Leaky-Integrator Striatum D1 "/1
  "Leaky-Integrator Striatum D1 "/1 -> "Sigmoidal Thalamus "/1
  "Sigmoidal Thalamus "/1 -> Out1/1

== system ExtensionSimulation2CONT/SMA 3/Memory/Self-Resetting System ==
  In1 : Inport
  Product : Product
  Relay : Relay  OnSwitchValue=MemoryGain  OffSwitchValue=0.1
  Reset Timer : Subsystem
  Saturation : Saturate
  Scope : Scope  NumInputPorts=2
  Out1 : Outport
  wires:
  Relay/1 -> Reset Timer/1(R)
  In1/1 -> Product/2, Scope/1, Relay/1
  Reset Timer/1(Out) -> Product/1
  Product/1 -> Saturation/1
  Saturation/1 -> Out1/1, Scope/2

== system ExtensionSimulation2CONT/SMA 3/Thalamus CH3 /Neural Integration Thalamus  (pc) ==
  In1 : Inport
  "Leaky-Integrator Striatum D1 " : ZeroPole  Zeros=[]  Poles=[-1/teta]  Gain=[1.5/teta]
  "Sigmoidal Thalamus " : fuzblock/Membership  Functions/Sigmoidal MF  a=alpha_thal  c=beta_thal
  Out1 : Outport
  wires:
  In1/1 -> "Leaky-Integrator Striatum D1 "/1
  "Leaky-Integrator Striatum D1 "/1 -> "Sigmoidal Thalamus "/1
  "Sigmoidal Thalamus "/1 -> Out1/1

== system ExtensionSimulation2CONT/SMA 4/Memory/Self-Resetting System ==
  In1 : Inport
  Product : Product
  Relay : Relay  OnSwitchValue=MemoryGain  OffSwitchValue=0.1
  Reset Timer : Subsystem
  Saturation : Saturate
  Scope : Scope  NumInputPorts=2
  Out1 : Outport
  wires:
  Relay/1 -> Reset Timer/1(R)
  In1/1 -> Product/2, Scope/1, Relay/1
  Reset Timer/1(Out) -> Product/1
  Product/1 -> Saturation/1
  Saturation/1 -> Out1/1, Scope/2

== system ExtensionSimulation2CONT/SMA 4/Thalamus CH4 /Neural Integration Thalamus  (pc) ==
  In1 : Inport
  "Leaky-Integrator Striatum D1 " : ZeroPole  Zeros=[]  Poles=[-1/teta]  Gain=[1.5/teta]
  "Sigmoidal Thalamus " : fuzblock/Membership  Functions/Sigmoidal MF  a=alpha_thal  c=beta_thal
  Out1 : Outport
  wires:
  In1/1 -> "Leaky-Integrator Striatum D1 "/1
  "Leaky-Integrator Striatum D1 "/1 -> "Sigmoidal Thalamus "/1
  "Sigmoidal Thalamus "/1 -> Out1/1

== system ExtensionSimulation2CONT/SMA 5/Memory/Self-Resetting System ==
  In1 : Inport
  Product : Product
  Relay : Relay  OnSwitchValue=MemoryGain  OffSwitchValue=0.1
  Reset Timer : Subsystem
  Saturation : Saturate
  Scope : Scope  NumInputPorts=2
  Out1 : Outport
  wires:
  Relay/1 -> Reset Timer/1(R)
  In1/1 -> Product/2, Scope/1, Relay/1
  Reset Timer/1(Out) -> Product/1
  Product/1 -> Saturation/1
  Saturation/1 -> Out1/1, Scope/2

== system ExtensionSimulation2CONT/SMA 5/Thalamus CH5 /Neural Integration Thalamus  (pc) ==
  In1 : Inport
  "Leaky-Integrator Striatum D1 " : ZeroPole  Zeros=[]  Poles=[-1/teta]  Gain=[1.5/teta]
  "Sigmoidal Thalamus " : fuzblock/Membership  Functions/Sigmoidal MF  a=alpha_thal  c=beta_thal
  Out1 : Outport
  wires:
  In1/1 -> "Leaky-Integrator Striatum D1 "/1
  "Leaky-Integrator Striatum D1 "/1 -> "Sigmoidal Thalamus "/1
  "Sigmoidal Thalamus "/1 -> Out1/1

== system ExtensionSimulation2CONT/BASAL GANGLIA WITH 5 CHANNELS COMPETITION/GPe/GPe CH1/GPeSat ==
  In1 : Inport
  "Leaky-Integrator Striatum D1 " : ZeroPole  Zeros=[]  Poles=[-1/teta]  Gain=[1.5/teta]
  Sigmoidal MF : fuzblock/Membership  Functions/Sigmoidal MF  a=alpha_gpe  c=beta_gpe
  Out1 : Outport
  wires:
  Sigmoidal MF/1 -> Out1/1
  "Leaky-Integrator Striatum D1 "/1 -> Sigmoidal MF/1
  In1/1 -> "Leaky-Integrator Striatum D1 "/1

== system ExtensionSimulation2CONT/BASAL GANGLIA WITH 5 CHANNELS COMPETITION/GPe/GPe CH1/GPeSat1 ==
  In1 : Inport
  "Leaky-Integrator Striatum D1 " : ZeroPole  Zeros=[]  Poles=[-1/teta]  Gain=[1.5/teta]
  Sigmoidal MF : fuzblock/Membership  Functions/Sigmoidal MF  a=alpha_gpe  c=beta_gpe
  Out1 : Outport
  wires:
  Sigmoidal MF/1 -> Out1/1
  "Leaky-Integrator Striatum D1 "/1 -> Sigmoidal MF/1
  In1/1 -> "Leaky-Integrator Striatum D1 "/1

== system ExtensionSimulation2CONT/BASAL GANGLIA WITH 5 CHANNELS COMPETITION/GPe/GPe CH1/GPeSat2 ==
  In1 : Inport
  "Leaky-Integrator Striatum D1 " : ZeroPole  Zeros=[]  Poles=[-1/teta]  Gain=[1.5/teta]
  Sigmoidal MF : fuzblock/Membership  Functions/Sigmoidal MF  a=alpha_gpe  c=beta_gpe
  Out1 : Outport
  wires:
  Sigmoidal MF/1 -> Out1/1
  "Leaky-Integrator Striatum D1 "/1 -> Sigmoidal MF/1
  In1/1 -> "Leaky-Integrator Striatum D1 "/1

== system ExtensionSimulation2CONT/BASAL GANGLIA WITH 5 CHANNELS COMPETITION/GPe/GPe CH1/GPeSat3 ==
  In1 : Inport
  "Leaky-Integrator Striatum D1 " : ZeroPole  Zeros=[]  Poles=[-1/teta]  Gain=[1.5/teta]
  Sigmoidal MF : fuzblock/Membership  Functions/Sigmoidal MF  a=alpha_gpe  c=beta_gpe
  Out1 : Outport
  wires:
  Sigmoidal MF/1 -> Out1/1
  "Leaky-Integrator Striatum D1 "/1 -> Sigmoidal MF/1
  In1/1 -> "Leaky-Integrator Striatum D1 "/1

== system ExtensionSimulation2CONT/BASAL GANGLIA WITH 5 CHANNELS COMPETITION/GPe/GPe CH1/GPeSat4 ==
  In1 : Inport
  "Leaky-Integrator Striatum D1 " : ZeroPole  Zeros=[]  Poles=[-1/teta]  Gain=[1.5/teta]
  Sigmoidal MF : fuzblock/Membership  Functions/Sigmoidal MF  a=alpha_gpe  c=beta_gpe
  Out1 : Outport
  wires:
  Sigmoidal MF/1 -> Out1/1
  "Leaky-Integrator Striatum D1 "/1 -> Sigmoidal MF/1
  In1/1 -> "Leaky-Integrator Striatum D1 "/1

== system ExtensionSimulation2CONT/BASAL GANGLIA WITH 5 CHANNELS COMPETITION/GPi/GPinternal/GPinternal ==
  In1 : Inport
  "Leaky-Integrator Striatum D1 " : ZeroPole  Zeros=[]  Poles=[-1/teta]  Gain=[1.5/teta]
  Sigmoidal MF : fuzblock/Membership  Functions/Sigmoidal MF  a=alpha_gpi  c=beta_gpi
  Out1 : Outport
  wires:
  Sigmoidal MF/1 -> Out1/1
  "Leaky-Integrator Striatum D1 "/1 -> Sigmoidal MF/1
  In1/1 -> "Leaky-Integrator Striatum D1 "/1

== system ExtensionSimulation2CONT/BASAL GANGLIA WITH 5 CHANNELS COMPETITION/GPi/GPinternal/GPinternal1 ==
  In1 : Inport
  "Leaky-Integrator Striatum D1 " : ZeroPole  Zeros=[]  Poles=[-1/teta]  Gain=[1.5/teta]
  Sigmoidal MF : fuzblock/Membership  Functions/Sigmoidal MF  a=alpha_gpi  c=beta_gpi
  Out1 : Outport
  wires:
  Sigmoidal MF/1 -> Out1/1
  "Leaky-Integrator Striatum D1 "/1 -> Sigmoidal MF/1
  In1/1 -> "Leaky-Integrator Striatum D1 "/1

== system ExtensionSimulation2CONT/BASAL GANGLIA WITH 5 CHANNELS COMPETITION/GPi/GPinternal/GPinternal2 ==
  In1 : Inport
  "Leaky-Integrator Striatum D1 " : ZeroPole  Zeros=[]  Poles=[-1/teta]  Gain=[1.5/teta]
  Sigmoidal MF : fuzblock/Membership  Functions/Sigmoidal MF  a=alpha_gpi  c=beta_gpi
  Out1 : Outport
  wires:
  Sigmoidal MF/1 -> Out1/1
  "Leaky-Integrator Striatum D1 "/1 -> Sigmoidal MF/1
  In1/1 -> "Leaky-Integrator Striatum D1 "/1

== system ExtensionSimulation2CONT/BASAL GANGLIA WITH 5 CHANNELS COMPETITION/GPi/GPinternal/GPinternal3 ==
  In1 : Inport
  "Leaky-Integrator Striatum D1 " : ZeroPole  Zeros=[]  Poles=[-1/teta]  Gain=[1.5/teta]
  Sigmoidal MF : fuzblock/Membership  Functions/Sigmoidal MF  a=alpha_gpi  c=beta_gpi
  Out1 : Outport
  wires:
  Sigmoidal MF/1 -> Out1/1
  "Leaky-Integrator Striatum D1 "/1 -> Sigmoidal MF/1
  In1/1 -> "Leaky-Integrator Striatum D1 "/1

== system ExtensionSimulation2CONT/BASAL GANGLIA WITH 5 CHANNELS COMPETITION/GPi/GPinternal/GPinternal4 ==
  In1 : Inport
  "Leaky-Integrator Striatum D1 " : ZeroPole  Zeros=[]  Poles=[-1/teta]  Gain=[1.5/teta]
  Sigmoidal MF : fuzblock/Membership  Functions/Sigmoidal MF  a=alpha_gpi  c=beta_gpi
  Out1 : Outport
  wires:
  Sigmoidal MF/1 -> Out1/1
  "Leaky-Integrator Striatum D1 "/1 -> Sigmoidal MF/1
  In1/1 -> "Leaky-Integrator Striatum D1 "/1

== system ExtensionSimulation2CONT/BASAL GANGLIA WITH 5 CHANNELS COMPETITION/Striatum D1 /Striatum D1 /StrSat ==
  In1 : Inport
  "Leaky-Integrator Striatum D1 " : ZeroPole  Zeros=[]  Poles=[-1/teta]  Gain=[1.5/teta]
  Sigmoidal MF : fuzblock/Membership  Functions/Sigmoidal MF  a=alpha_str(1)  c=beta_str(1)
  Out1 : Outport
  wires:
  Sigmoidal MF/1 -> Out1/1
  "Leaky-Integrator Striatum D1 "/1 -> Sigmoidal MF/1
  In1/1 -> "Leaky-Integrator Striatum D1 "/1

== system ExtensionSimulation2CONT/BASAL GANGLIA WITH 5 CHANNELS COMPETITION/Striatum D1 /Striatum D1 /StrSat1 ==
  In1 : Inport
  "Leaky-Integrator Striatum D1 " : ZeroPole  Zeros=[]  Poles=[-1/teta]  Gain=[1.5/teta]
  Sigmoidal MF : fuzblock/Membership  Functions/Sigmoidal MF  a=alpha_str(2)  c=beta_str(2)
  Out1 : Outport
  wires:
  Sigmoidal MF/1 -> Out1/1
  "Leaky-Integrator Striatum D1 "/1 -> Sigmoidal MF/1
  In1/1 -> "Leaky-Integrator Striatum D1 "/1

== system ExtensionSimulation2CONT/BASAL GANGLIA WITH 5 CHANNELS COMPETITION/Striatum D1 /Striatum D1 /StrSat2 ==
  In1 : Inport
  "Leaky-Integrator Striatum D1 " : ZeroPole  Zeros=[]  Poles=[-1/teta]  Gain=[1.5/teta]
  Sigmoidal MF : fuzblock/Membership  Functions/Sigmoidal MF  a=alpha_str(3)  c=beta_str(3)
  Out1 : Outport
  wires:
  Sigmoidal MF/1 -> Out1/1
  "Leaky-Integrator Striatum D1 "/1 -> Sigmoidal MF/1
  In1/1 -> "Leaky-Integrator Striatum D1 "/1

== system ExtensionSimulation2CONT/BASAL GANGLIA WITH 5 CHANNELS COMPETITION/Striatum D1 /Striatum D1 /StrSat3 ==
  In1 : Inport
  "Leaky-Integrator Striatum D1 " : ZeroPole  Zeros=[]  Poles=[-1/teta]  Gain=[1.5/teta]
  Sigmoidal MF : fuzblock/Membership  Functions/Sigmoidal MF  a=alpha_str(4)  c=beta_str(4)
  Out1 : Outport
  wires:
  Sigmoidal MF/1 -> Out1/1
  "Leaky-Integrator Striatum D1 "/1 -> Sigmoidal MF/1
  In1/1 -> "Leaky-Integrator Striatum D1 "/1

== system ExtensionSimulation2CONT/BASAL GANGLIA WITH 5 CHANNELS COMPETITION/Striatum D1 /Striatum D1 /StrSat4 ==
  In1 : Inport
  "Leaky-Integrator Striatum D1 " : ZeroPole  Zeros=[]  Poles=[-1/teta]  Gain=[1.5/teta]
  Sigmoidal MF : fuzblock/Membership  Functions/Sigmoidal MF  a=alpha_str(5)  c=beta_str(5)
  Out1 : Outport
  wires:
  Sigmoidal MF/1 -> Out1/1
  "Leaky-Integrator Striatum D1 "/1 -> Sigmoidal MF/1
  In1/1 -> "Leaky-Integrator Striatum D1 "/1

== system ExtensionSimulation2CONT/BASAL GANGLIA WITH 5 CHANNELS COMPETITION/Striatum D2/Striatum D2 /StrSat ==
  In1 : Inport
  "Leaky-Integrator Striatum D1 " : ZeroPole  Zeros=[]  Poles=[-1/teta]  Gain=[1.5/teta]
  Sigmoidal MF : fuzblock/Membership  Functions/Sigmoidal MF  a=alpha_str(1)  c=beta_str(1)
  Out1 : Outport
  wires:
  Sigmoidal MF/1 -> Out1/1
  "Leaky-Integrator Striatum D1 "/1 -> Sigmoidal MF/1
  In1/1 -> "Leaky-Integrator Striatum D1 "/1

== system ExtensionSimulation2CONT/BASAL GANGLIA WITH 5 CHANNELS COMPETITION/Striatum D2/Striatum D2 /StrSat1 ==
  In1 : Inport
  "Leaky-Integrator Striatum D1 " : ZeroPole  Zeros=[]  Poles=[-1/teta]  Gain=[1.5/teta]
  Sigmoidal MF : fuzblock/Membership  Functions/Sigmoidal MF  a=alpha_str(2)  c=beta_str(2)
  Out1 : Outport
  wires:
  Sigmoidal MF/1 -> Out1/1
  "Leaky-Integrator Striatum D1 "/1 -> Sigmoidal MF/1
  In1/1 -> "Leaky-Integrator Striatum D1 "/1

== system ExtensionSimulation2CONT/BASAL GANGLIA WITH 5 CHANNELS COMPETITION/Striatum D2/Striatum D2 /StrSat2 ==
  In1 : Inport
  "Leaky-Integrator Striatum D1 " : ZeroPole  Zeros=[]  Poles=[-1/teta]  Gain=[1.5/teta]
  Sigmoidal MF : fuzblock/Membership  Functions/Sigmoidal MF  a=alpha_str(3)  c=beta_str(3)
  Out1 : Outport
  wires:
  Sigmoidal MF/1 -> Out1/1
  "Leaky-Integrator Striatum D1 "/1 -> Sigmoidal MF/1
  In1/1 -> "Leaky-Integrator Striatum D1 "/1

== system ExtensionSimulation2CONT/BASAL GANGLIA WITH 5 CHANNELS COMPETITION/Striatum D2/Striatum D2 /StrSat3 ==
  In1 : Inport
  "Leaky-Integrator Striatum D1 " : ZeroPole  Zeros=[]  Poles=[-1/teta]  Gain=[1.5/teta]
  Sigmoidal MF : fuzblock/Membership  Functions/Sigmoidal MF  a=alpha_str(4)  c=beta_str(4)
  Out1 : Outport
  wires:
  Sigmoidal MF/1 -> Out1/1
  "Leaky-Integrator Striatum D1 "/1 -> Sigmoidal MF/1
  In1/1 -> "Leaky-Integrator Striatum D1 "/1

== system ExtensionSimulation2CONT/BASAL GANGLIA WITH 5 CHANNELS COMPETITION/Striatum D2/Striatum D2 /StrSat4 ==
  In1 : Inport
  "Leaky-Integrator Striatum D1 " : ZeroPole  Zeros=[]  Poles=[-1/teta]  Gain=[1.5/teta]
  Sigmoidal MF : fuzblock/Membership  Functions/Sigmoidal MF  a=alpha_str(5)  c=beta_str(5)
  Out1 : Outport
  wires:
  Sigmoidal MF/1 -> Out1/1
  "Leaky-Integrator Striatum D1 "/1 -> Sigmoidal MF/1
  In1/1 -> "Leaky-Integrator Striatum D1 "/1

== system ExtensionSimulation2CONT/BASAL GANGLIA WITH 5 CHANNELS COMPETITION/SubThalamic Nuclei/SubThalamic Nucleus (STN) /StnSat ==
  In1 : Inport
  "Leaky-Integrator Striatum D1 " : ZeroPole  Zeros=[]  Poles=[-1/teta]  Gain=[1.5/teta]
  Sigmoidal MF : fuzblock/Membership  Functions/Sigmoidal MF  a=alpha_stn  c=beta_stn
  Out1 : Outport
  wires:
  Sigmoidal MF/1 -> Out1/1
  "Leaky-Integrator Striatum D1 "/1 -> Sigmoidal MF/1
  In1/1 -> "Leaky-Integrator Striatum D1 "/1

== system ExtensionSimulation2CONT/BASAL GANGLIA WITH 5 CHANNELS COMPETITION/SubThalamic Nuclei/SubThalamic Nucleus (STN) /StnSat1 ==
  In1 : Inport
  "Leaky-Integrator Striatum D1 " : ZeroPole  Zeros=[]  Poles=[-1/teta]  Gain=[1.5/teta]
  Sigmoidal MF : fuzblock/Membership  Functions/Sigmoidal MF  a=alpha_stn  c=beta_stn
  Out1 : Outport
  wires:
  Sigmoidal MF/1 -> Out1/1
  "Leaky-Integrator Striatum D1 "/1 -> Sigmoidal MF/1
  In1/1 -> "Leaky-Integrator Striatum D1 "/1

== system ExtensionSimulation2CONT/BASAL GANGLIA WITH 5 CHANNELS COMPETITION/SubThalamic Nuclei/SubThalamic Nucleus (STN) /StnSat2 ==
  In1 : Inport
  "Leaky-Integrator Striatum D1 " : ZeroPole  Zeros=[]  Poles=[-1/teta]  Gain=[1.5/teta]
  Sigmoidal MF : fuzblock/Membership  Functions/Sigmoidal MF  a=alpha_stn  c=beta_stn
  Out1 : Outport
  wires:
  Sigmoidal MF/1 -> Out1/1
  "Leaky-Integrator Striatum D1 "/1 -> Sigmoidal MF/1
  In1/1 -> "Leaky-Integrator Striatum D1 "/1

== system ExtensionSimulation2CONT/BASAL GANGLIA WITH 5 CHANNELS COMPETITION/SubThalamic Nuclei/SubThalamic Nucleus (STN) /StnSat3 ==
  In1 : Inport
  "Leaky-Integrator Striatum D1 " : ZeroPole  Zeros=[]  Poles=[-1/teta]  Gain=[1.5/teta]
  Sigmoidal MF : fuzblock/Membership  Functions/Sigmoidal MF  a=alpha_stn  c=beta_stn
  Out1 : Outport
  wires:
  Sigmoidal MF/1 -> Out1/1
  "Leaky-Integrator Striatum D1 "/1 -> Sigmoidal MF/1
  In1/1 -> "Leaky-Integrator Striatum D1 "/1

== system ExtensionSimulation2CONT/BASAL GANGLIA WITH 5 CHANNELS COMPETITION/SubThalamic Nuclei/SubThalamic Nucleus (STN) /StnSat4 ==
  In1 : Inport
  "Leaky-Integrator Striatum D1 " : ZeroPole  Zeros=[]  Poles=[-1/teta]  Gain=[1.5/teta]
  Sigmoidal MF : fuzblock/Membership  Functions/Sigmoidal MF  a=alpha_stn  c=beta_stn
  Out1 : Outport
  wires:
  Sigmoidal MF/1 -> Out1/1
  "Leaky-Integrator Striatum D1 "/1 -> Sigmoidal MF/1
  In1/1 -> "Leaky-Integrator Striatum D1 "/1

== system ExtensionSimulation2CONT/SMA 1/Memory/Self-Resetting System/Reset Timer ==
  R : Inport
  Clock1 : Clock
  Clock3 : Clock
      settings: Decimation=4
  Sum1 : Sum  Inputs=|+-  SaturateOnIntegerOverflow=on  InputSameDT=on  OutDataTypeStr=Inherit: Same as first input
  Switch2 : Switch  Threshold=1  RndMeth=Zero
  Out : Outport
  wires:
  Clock1/1 -> Sum1/1
  Clock3/1 -> Switch2/3
  Switch2/1 -> Switch2/1, Sum1/2
  Sum1/1 -> Out/1
  R/1 -> Switch2/2

== system ExtensionSimulation2CONT/SMA 2/Memory/Self-Resetting System/Reset Timer ==
  R : Inport
  Clock1 : Clock
  Clock3 : Clock
      settings: Decimation=4
  Sum1 : Sum  Inputs=|+-  SaturateOnIntegerOverflow=on  InputSameDT=on  OutDataTypeStr=Inherit: Same as first input
  Switch2 : Switch  Threshold=1  RndMeth=Zero
  Out : Outport
  wires:
  Clock1/1 -> Sum1/1
  Clock3/1 -> Switch2/3
  Switch2/1 -> Switch2/1, Sum1/2
  Sum1/1 -> Out/1
  R/1 -> Switch2/2

== system ExtensionSimulation2CONT/SMA 3/Memory/Self-Resetting System/Reset Timer ==
  R : Inport
  Clock1 : Clock
  Clock3 : Clock
      settings: Decimation=4
  Sum1 : Sum  Inputs=|+-  SaturateOnIntegerOverflow=on  InputSameDT=on  OutDataTypeStr=Inherit: Same as first input
  Switch2 : Switch  Threshold=1  RndMeth=Zero
  Out : Outport
  wires:
  Clock1/1 -> Sum1/1
  Clock3/1 -> Switch2/3
  Switch2/1 -> Switch2/1, Sum1/2
  Sum1/1 -> Out/1
  R/1 -> Switch2/2

== system ExtensionSimulation2CONT/SMA 4/Memory/Self-Resetting System/Reset Timer ==
  R : Inport
  Clock1 : Clock
  Clock3 : Clock
      settings: Decimation=4
  Sum1 : Sum  Inputs=|+-  SaturateOnIntegerOverflow=on  InputSameDT=on  OutDataTypeStr=Inherit: Same as first input
  Switch2 : Switch  Threshold=1  RndMeth=Zero
  Out : Outport
  wires:
  Clock1/1 -> Sum1/1
  Clock3/1 -> Switch2/3
  Switch2/1 -> Switch2/1, Sum1/2
  Sum1/1 -> Out/1
  R/1 -> Switch2/2

== system ExtensionSimulation2CONT/SMA 5/Memory/Self-Resetting System/Reset Timer ==
  R : Inport
  Clock1 : Clock
  Clock3 : Clock
      settings: Decimation=4
  Sum1 : Sum  Inputs=|+-  SaturateOnIntegerOverflow=on  InputSameDT=on  OutDataTypeStr=Inherit: Same as first input
  Switch2 : Switch  Threshold=1  RndMeth=Zero
  Out : Outport
  wires:
  Clock1/1 -> Sum1/1
  Clock3/1 -> Switch2/3
  Switch2/1 -> Switch2/1, Sum1/2
  Sum1/1 -> Out/1
  R/1 -> Switch2/2
